simulink model "model"  (Simulink 7.9)
settings: Solver=ode45  StartTime=0.0  StopTime=10  RelTol=1e-3
values from neighbouring files (symbols this model uses):
  c_B = param(2)    [TF_acc.m]    (also in TF_fdyn.m; bode_plot.m; para.m = 20000)
  c_W = param(5)    [TF_acc.m]    (also in TF_fdyn.m; bode_plot.m; para.m = 150000)
  d_B = param(3)    [TF_acc.m]    (also in TF_fdyn.m; bode_plot.m; para.m = 1500)
  d_W = param(6)    [TF_acc.m]    (also in TF_fdyn.m; bode_plot.m; para.m = 100)
  f = 50    [bodydamping_var.m]    (also in bodymass_var.m; bodystiffness_var.m; tirestiffness_var.m; wheelmass_var.m = freq(i))
  m_B = param(1)    [TF_acc.m]    (also in TF_fdyn.m; bode_plot.m; para.m = 400)
  m_W = param(4)    [TF_acc.m]    (also in TF_fdyn.m; bode_plot.m; para.m = 50; wheelmass_var.m = wheelmass(h))
settings Model: Creator=DN  LastModifiedBy=DN

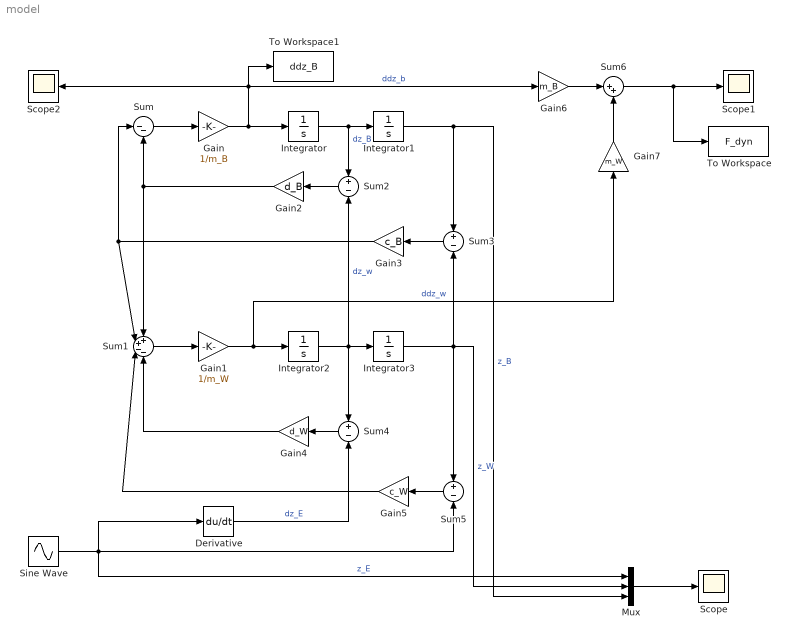
== system model ==
  Derivative : Derivative
  Gain : Gain  Gain=1/m_B
  Gain1 : Gain  Gain=1/m_W
  Gain2 : Gain  Gain=d_B
  Gain3 : Gain  Gain=c_B
  Gain4 : Gain  Gain=d_W
  Gain5 : Gain  Gain=c_W
  Gain6 : Gain  Gain=m_B
  Gain7 : Gain  Gain=m_W
  Integrator{,1..3} (4 alike) : Integrator
  Mux : Mux  Inputs=3
  Scope : Scope
  Scope1 : Scope
  Scope2 : Scope
      settings: SaveName=ScopeData2
  Sine Wave : Sin  Amplitude=0.1  Frequency=f*2*pi  SampleTime=0
  Sum : Sum  Inputs=|--
  Sum1 : Sum  Inputs=++--
  Sum{2..5} (4 alike) : Sum  Inputs=+|-
  Sum6 : Sum  Inputs=|++
  To Workspace : ToWorkspace  VariableName=F_dyn  SampleTime=-1
  To Workspace1 : ToWorkspace  VariableName=ddz_B  SampleTime=-1
  wires:
  Sum/1 -> Gain/1
  Gain/1 -> Integrator/1, Gain6/1, Scope2/1, To Workspace1/1  "ddz_b"
  Integrator/1 -> Integrator1/1, Sum2/1  "dz_B"
  Sum1/1 -> Gain1/1
  Gain1/1 -> Integrator2/1, Gain7/1  "ddz_w"
  Integrator2/1 -> Integrator3/1, Sum2/2, Sum4/1  "dz_w"
  Sum2/1 -> Gain2/1
  Gain2/1 -> Sum/2, Sum1/1
  Integrator1/1 -> Sum3/1, Mux/3  "z_B"
  Integrator3/1 -> Sum3/2, Sum5/1, Mux/2  "z_W"
  Sum3/1 -> Gain3/1
  Gain3/1 -> Sum/1, Sum1/2
  Sine Wave/1 -> Mux/1, Sum5/2, Derivative/1  "z_E"
  Sum4/1 -> Gain4/1
  Gain4/1 -> Sum1/4
  Sum5/1 -> Gain5/1
  Mux/1 -> Scope/1
  Gain5/1 -> Sum1/3
  Derivative/1 -> Sum4/2  "dz_E"
  Gain6/1 -> Sum6/1
  Gain7/1 -> Sum6/2
  Sum6/1 -> Scope1/1, To Workspace/1
